simulink model "simulink_problem_2_7_97"  (R2017b)
settings: Solver=VariableStepAuto  StartTime=0.0  StopTime=10.0  RelTol=1e-3
settings Model: Creator=ghost  LastModifiedBy=ghost

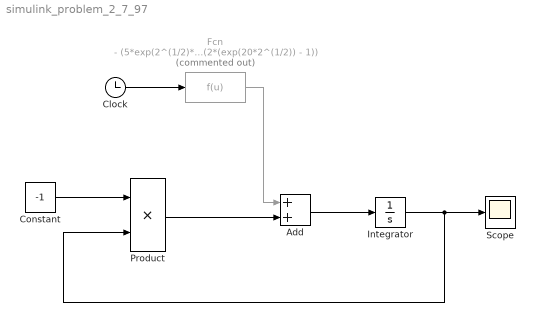
== system simulink_problem_2_7_97 ==
  Add : Sum
  Clock : Clock
  Constant : Constant  Value=-1
  Fcn : Fcn  Commented=on  Expr=- (5*exp(2^(1/2)*u)*(2*2^(1/2) + 2))/(2*(exp(20*2^(1/2)) - 1)) - (5*exp(20*2^(1/2))*exp(-2^(1/2)*u)*(2*2^(1/2) - 2))/(2*(exp(20*2^(1/2)) - 1))
  Integrator : Integrator  InitialCondition=5
  Product : Product
  Scope : Scope
  wires:
  Constant/1 -> Product/1
  Integrator/1 -> Product/2, Scope/1
  Add/1 -> Integrator/1
  Product/1 -> Add/2
  Clock/1 -> Fcn/1
  Fcn/1 -> Add/1
